simulink library "lib_ofdmrx"  (R2020a)
settings: Solver=VariableStepAuto  StartTime=0.0  StopTime=10.0  RelTol=1e-3
undefined symbols (not defined in the file): fs, LTSfreq, pilot, read_addr_rx, sc_index
libraries: simulink x36, hdlsllib x27, dsphdlmathfun x3, dspsigops x2, dsphdlxfrm x1, dsphdlsigops x1
(part 3 of 3)

== system lib_ofdmrx/OFDMRx/Synchronisation/SchmidlCoxMetric /CIC_ma ==
  note: The averaging window is set to 64 samples i.e.
      | 4x repetitions of the L-STF. Using a larger averaging
      | window improves the coarse CFO estimate. This
      | approach leaves 6x L-STF repetitions for AGC convergence.
  In1 : Inport
  Add : Sum  Inputs=-+  AccumDataTypeStr=fixdt(1,33,23)
  Add1 : Sum  AccumDataTypeStr=fixdt(1,33,23)
  Data Type Conversion : DataTypeConversion  OutDataTypeStr=fixdt(1,18,16)
  Delay1 : Delay  DelayLength=48
  Delay2 : Delay  DelayLength=1
  Delay3 : Delay  DelayLength=1
  Delay4 : Delay  DelayLength=1
  Out1 : Outport  VectorParamsAs1DForOutWhenUnconnected=off
  wires:
  Add/1 -> Add1/2
  Delay1/1 -> Add/1
  In1/1 -> Delay3/1
  Add1/1 -> Delay2/1
  Delay2/1 -> Delay4/1, Add1/1
  Delay3/1 -> Add/2, Delay1/1
  Delay4/1 -> Data Type Conversion/1
  Data Type Conversion/1 -> Out1/1

== system lib_ofdmrx/OFDMRx/Synchronisation/SchmidlCoxMetric /CIC_ma1 ==
  In1 : Inport
  Add : Sum  Inputs=-+  AccumDataTypeStr=fixdt(1,33,23)
  Add1 : Sum  AccumDataTypeStr=fixdt(1,33,23)
  Data Type Conversion : DataTypeConversion  OutDataTypeStr=fixdt(1,18,15)
  Delay1 : Delay  DelayLength=48
  Delay2 : Delay  DelayLength=1
  Delay3 : Delay  DelayLength=1
  Delay4 : Delay  DelayLength=1
  Out1 : Outport  VectorParamsAs1DForOutWhenUnconnected=off
  wires:
  Delay2/1 -> Add1/1, Delay4/1
  Add1/1 -> Delay2/1
  In1/1 -> Delay3/1
  Delay1/1 -> Add/1
  Add/1 -> Add1/2
  Delay3/1 -> Delay1/1, Add/2
  Delay4/1 -> Data Type Conversion/1
  Data Type Conversion/1 -> Out1/1

== system lib_ofdmrx/OFDMRx/Synchronisation/SchmidlCoxMetric /MagPhase ==
  dataIn : Inport
  Complex to Magnitude-Angle HDL Optimized : dsphdlmathfun/Complex to Magnitude-Angle HDL Optimized  NumIterationsSource=Property  NumIterations=10  OutputFormat=Magnitude and angle  AngleFormat=Normalized  ScaleOutput=on  SimulateUsing=Code generation
      settings: SourceProductBaseCode=DS
  Constant : Constant  OutDataTypeStr=boolean  SampleTime=1/fs
  Data Type Conversion : DataTypeConversion  OutDataTypeStr=fixdt(1,18,16)
  Data Type Conversion1 : DataTypeConversion  OutDataTypeStr=fixdt(1,25,22)
  Terminator1 : Terminator
  Phase : Outport  VectorParamsAs1DForOutWhenUnconnected=off
  Mag : Outport  Port=2  VectorParamsAs1DForOutWhenUnconnected=off
  wires:
  Constant/1 -> Complex to Magnitude-Angle HDL Optimized/2
  dataIn/1 -> Complex to Magnitude-Angle HDL Optimized/1
  Complex to Magnitude-Angle HDL Optimized/1 -> Data Type Conversion/1
  Complex to Magnitude-Angle HDL Optimized/3 -> Terminator1/1
  Complex to Magnitude-Angle HDL Optimized/2 -> Data Type Conversion1/1
  Data Type Conversion/1 -> Mag/1
  Data Type Conversion1/1 -> Phase/1

== system lib_ofdmrx/OFDMRx/Synchronisation/SchmidlCoxMetric /Sq ==
  In1 : Inport
  Delay : Delay  DelayLength=1
  Delay1 : Delay  DelayLength=1
  Product : Product
  Out1 : Outport  VectorParamsAs1DForOutWhenUnconnected=off
  wires:
  In1/1 -> Delay/1
  Product/1 -> Delay1/1
  Delay/1 -> Product/1, Product/2
  Delay1/1 -> Out1/1

== system lib_ofdmrx/OFDMRx/Synchronisation/SchmidlCoxMetric /Sq1 ==
  In1 : Inport
  Delay : Delay  DelayLength=1
  Delay1 : Delay  DelayLength=1
  Product : Product
  Out1 : Outport  VectorParamsAs1DForOutWhenUnconnected=off
  wires:
  Delay1/1 -> Out1/1
  Delay/1 -> Product/2, Product/1
  Product/1 -> Delay1/1
  In1/1 -> Delay/1

== system lib_ofdmrx/OFDMRx/Synchronisation/SchmidlCoxMetric /ThreshMult ==
  In1 : Inport
  ThreshMult : Gain  Gain=0.5  OutDataTypeStr=fixdt(1,33,23)
  Out1 : Outport  VectorParamsAs1DForOutWhenUnconnected=off
  wires:
  ThreshMult/1 -> Out1/1
  In1/1 -> ThreshMult/1

== system lib_ofdmrx/OFDMRx/PhaseTracking_1/PilotCtrlGen/pilotGen/ToComplex1 ==
  In1 : Inport
  Constant1 : Constant  Value=0  OutDataTypeStr=fixdt(1,2,0)  SampleTime=1/fs
  Real-Imag to Complex : RealImagToComplex
  Out1 : Outport  VectorParamsAs1DForOutWhenUnconnected=off
  wires:
  Constant1/1 -> Real-Imag to Complex/2
  In1/1 -> Real-Imag to Complex/1
  Real-Imag to Complex/1 -> Out1/1

== system lib_ofdmrx/OFDMRx/PhaseTracking_2/PilotCtrlGen/pilotGen/ToComplex1 ==
  In1 : Inport
  Constant1 : Constant  Value=0  OutDataTypeStr=fixdt(1,2,0)  SampleTime=1/fs
  Real-Imag to Complex : RealImagToComplex
  Out1 : Outport  VectorParamsAs1DForOutWhenUnconnected=off
  wires:
  Constant1/1 -> Real-Imag to Complex/2
  In1/1 -> Real-Imag to Complex/1
  Real-Imag to Complex/1 -> Out1/1

== system lib_ofdmrx/OFDMRx/Synchronisation/ControlSigGen/PreambleValidGen/RisingEdge ==
  ValidIn : Inport
  Delay : Delay  DelayLength=1
  Relational Operator : RelationalOperator  Operator=>  OutDataTypeStr=boolean  RndMeth=Nearest
  Out1 : Outport
  wires:
  ValidIn/1 -> Relational Operator/1, Delay/1
  Delay/1 -> Relational Operator/2
  Relational Operator/1 -> Out1/1

== matlab function lib_ofdmrx/OFDMRx/PhaseTracking_1/CordicRotate/QCORR/QUAD_MAP1 ==
  data: xin input; xout output; yout output; yin input; ctrl input
function [xout,yout] = fcn(xin,yin,ctrl)
% Process to perform final rotation 
% by pi/2 if the original angle was 
% in 3rd or 4th quadrants    
if ctrl == 0
    % 1st or 2nd quadrants 
    xout = fi(xin,1,21,15);  
    yout = fi(yin,1,21,15);  
elseif ctrl == 1
    % 3rd quadrant (rotate pi/2 clockwise)
    xout = fi(yin,1,21,15); 
    yout = fi(-xin,1,21,15); 
elseif ctrl == 2
    % 4th quadrant (rotate pi/2 anti-clockwise) 
    xout = fi(-yin,1,21,15); 
    yout = fi(xin,1,21,15); 
else 
    % others clause
    xout = fi(xin,1,21,15); 
    yout = fi(yin,1,21,15); 
end

== matlab function lib_ofdmrx/OFDMRx/PhaseTracking_1/CordicRotate/QUAD_MAP/QUAD_DETERM1 ==
  data: ang_in input; ang_out output; QUAD output
function [ang_out,QUAD] = fcn(ang_in)
% Process to determine quadrant and 
% shift into region -pi/2 to pi/2 if 
% not already there 
v = fi(pi,1,23,20);
x = fi(-pi,1,23,20); 
y = fi(-pi/2,1,23,20); 
z = fi(pi/2,1,23,20);

% Determine quadrant 
if ((ang_in >= y) && (ang_in <= z))
    QUAD = fi(0,0,2,0); % Quads 1 or 2
elseif ((ang_in < y) && (ang_in >= x))
    QUAD = fi(1,0,2,0); % Quad 3
elseif ((ang_in > z) && (ang_in <= v))
    QUAD = fi(2,0,2,0); % Quad 4
else 
    % others clause
    QUAD = fi(0,0,2,0);
end 

% Determine whether we need to add or subtract pi/2 
% based on quadrant location
switch(QUAD) 
    
    case 0 
        % Angle stays the same 
        ang_out = fi(ang_in, 1, 23, 20); 
    case 1
        % pi/2 is added to angle (anti-clockwise)
        ang_out = fi(ang_in + z, 1, 23, 20); 
    case 2
        % pi/2 is subtracted from angle (clockwise)
        ang_out = fi(ang_in - z, 1, 23, 20); 
    otherwise
        % others clause make output angle 
        % equal to input angle  
        ang_out = fi(ang_in, 1, 23, 20); 
end

== matlab function lib_ofdmrx/OFDMRx/PhaseTracking_2/CordicRotate/QCORR/QUAD_MAP1 ==
  data: xin input; xout output; yout output; yin input; ctrl input
function [xout,yout] = fcn(xin,yin,ctrl)
% Process to perform final rotation 
% by pi/2 if the original angle was 
% in 3rd or 4th quadrants    
if ctrl == 0
    % 1st or 2nd quadrants 
    xout = fi(xin,1,21,15);  
    yout = fi(yin,1,21,15);  
elseif ctrl == 1
    % 3rd quadrant (rotate pi/2 clockwise)
    xout = fi(yin,1,21,15); 
    yout = fi(-xin,1,21,15); 
elseif ctrl == 2
    % 4th quadrant (rotate pi/2 anti-clockwise) 
    xout = fi(-yin,1,21,15); 
    yout = fi(xin,1,21,15); 
else 
    % others clause
    xout = fi(xin,1,21,15); 
    yout = fi(yin,1,21,15); 
end

== matlab function lib_ofdmrx/OFDMRx/PhaseTracking_2/CordicRotate/QUAD_MAP/QUAD_DETERM1 ==
  data: ang_in input; ang_out output; QUAD output
function [ang_out,QUAD] = fcn(ang_in)
% Process to determine quadrant and 
% shift into region -pi/2 to pi/2 if 
% not already there 
v = fi(pi,1,23,20);
x = fi(-pi,1,23,20); 
y = fi(-pi/2,1,23,20); 
z = fi(pi/2,1,23,20);

% Determine quadrant 
if ((ang_in >= y) && (ang_in <= z))
    QUAD = fi(0,0,2,0); % Quads 1 or 2
elseif ((ang_in < y) && (ang_in >= x))
    QUAD = fi(1,0,2,0); % Quad 3
elseif ((ang_in > z) && (ang_in <= v))
    QUAD = fi(2,0,2,0); % Quad 4
else 
    % others clause
    QUAD = fi(0,0,2,0);
end 

% Determine whether we need to add or subtract pi/2 
% based on quadrant location
switch(QUAD) 
    
    case 0 
        % Angle stays the same 
        ang_out = fi(ang_in, 1, 23, 20); 
    case 1
        % pi/2 is added to angle (anti-clockwise)
        ang_out = fi(ang_in + z, 1, 23, 20); 
    case 2
        % pi/2 is subtracted from angle (clockwise)
        ang_out = fi(ang_in - z, 1, 23, 20); 
    otherwise
        % others clause make output angle 
        % equal to input angle  
        ang_out = fi(ang_in, 1, 23, 20); 
end
